simulink model "GNC_integrated_with_guidance"  (R2023a)
settings: Solver=VariableStepAuto  StartTime=0.0  StopTime=200  RelTol=1e-3
undefined symbols (not defined in the file or in its folder): param
libraries: eeGeneralControl x12, simulink_extras x6, SignalEditorBlockLib x1, sharedTrackingLibrary x1
settings Model: Creator=timme  LastModifiedBy=jipva

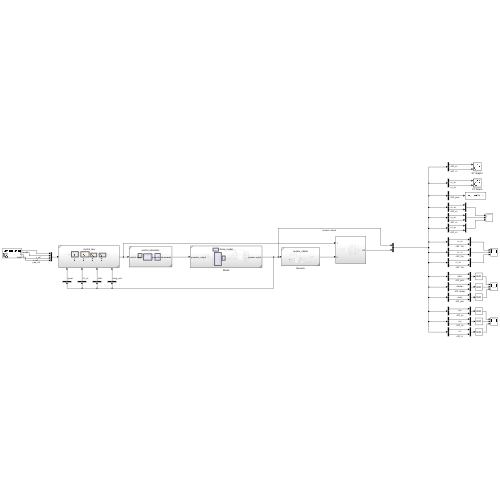
[thumbnail: Simulink's stored preview of the top-level diagram]
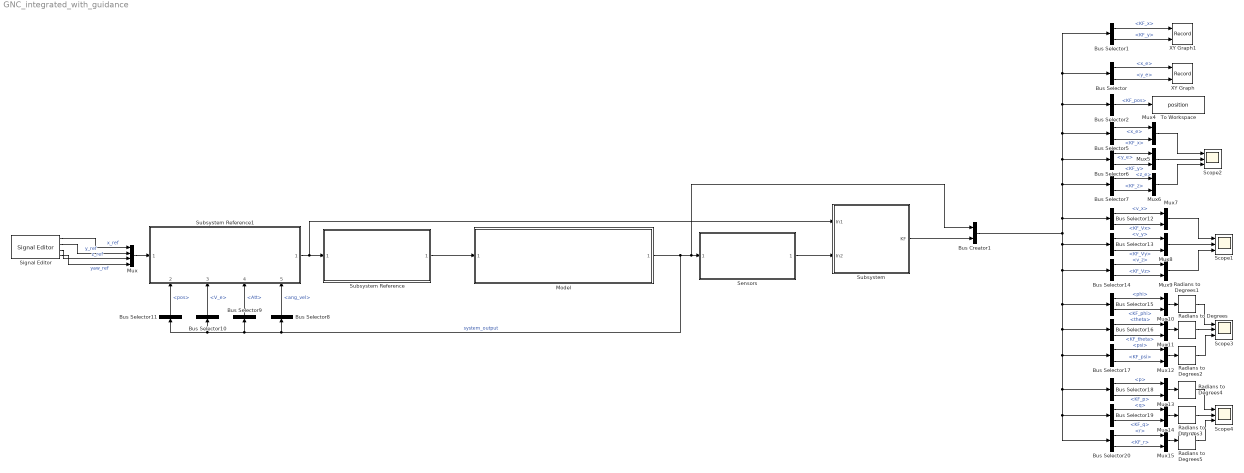
== system GNC_integrated_with_guidance ==
  Bus Creator1 : BusCreator  Inputs=2
  Bus Selector : BusSelector  OutputSignals=system_output.pos.x_e,system_output.pos.y_e
  Bus Selector1 : BusSelector  OutputSignals=KF.KF_pos.KF_x,KF.KF_pos.KF_y
  Bus Selector10 : BusSelector  OutputSignals=V_e
  Bus Selector11 : BusSelector  OutputSignals=pos
  Bus Selector12 : BusSelector  OutputSignals=system_output.V_e.v_x,KF.KF_vel.KF_Vx
  Bus Selector13 : BusSelector  OutputSignals=system_output.V_e.v_y,KF.KF_vel.KF_Vy
  Bus Selector14 : BusSelector  OutputSignals=system_output.V_e.v_z,KF.KF_vel.KF_Vz
  Bus Selector15 : BusSelector  OutputSignals=system_output.Att.phi,KF.KF_att.KF_phi
  Bus Selector16 : BusSelector  OutputSignals=system_output.Att.theta,KF.KF_att.KF_theta
  Bus Selector17 : BusSelector  OutputSignals=system_output.Att.psi,KF.KF_att.KF_psi
  Bus Selector18 : BusSelector  OutputSignals=system_output.ang_vel.p,KF.KF_omega.KF_p
  Bus Selector19 : BusSelector  OutputSignals=system_output.ang_vel.q,KF.KF_omega.KF_q
  Bus Selector2 : BusSelector  OutputSignals=KF.KF_pos
  Bus Selector20 : BusSelector  OutputSignals=system_output.ang_vel.r,KF.KF_omega.KF_r
  Bus Selector5 : BusSelector  OutputSignals=system_output.pos.x_e,KF.KF_pos.KF_x
  Bus Selector6 : BusSelector  OutputSignals=system_output.pos.y_e,KF.KF_pos.KF_y
  Bus Selector7 : BusSelector  OutputSignals=system_output.pos.z_e,KF.KF_pos.KF_z
  Bus Selector8 : BusSelector  OutputSignals=ang_vel
  Bus Selector9 : BusSelector  OutputSignals=Att
  Model : Subsystem  ReferencedSubsystem=drone_model
  Mux : Mux
  Mux{4..15} (12 alike) : Mux  Inputs=2
  Radians to Degrees{,1..5} (6 alike) : simulink_extras/Transformations/Radians to Degrees
  Scope{1..4} (4 alike) : Scope  NumInputPorts=3
  Sensors : Subsystem  ReferencedSubsystem=sensor_model
  Signal Editor : SignalEditorBlockLib/Signal Editor  FileName=C:\Users\jipva\MATLAB\Projects\drone\Detailed design phase\guidance\full_system_reference.mat  ActiveScenario=StandardScenario  ActiveSignal=yaw  IsBus=off  OutputBusObjectStr=Bus: BusObject  SampleTime=param.dt  ZeroCross=off  OutputAfterFinalValue=Setting to zero  Unit=inherit  PreserveSignalName=on  ApplySigPropsToAllScenarios=on
  Subsystem : Subsystem
  Subsystem Reference : Subsystem  ReferencedSubsystem=control_allocation
  Subsystem Reference1 : Subsystem  ReferencedSubsystem=control_law
      settings: PortSchema="{\"entries\":[{\"content\":{\"sides\":[{\"content\":{\"connectorIds\":[\"In1\"]},\"type\":\"ConnectorPlacement.EquallySpacedRectSide\",\"uuid\":\"cbb659e7-d19a-4e68-9ae7-e5e39426296b\"},{\"content\":{\"connectorIds\":[\"Out1\"],\"side\":\"RIGHT\"},\"type\":\"ConnectorPlacement.EquallySpacedRectSide\",\"uuid\":\"c9f08a4e-80d9-41bf-93e6-4cfd11b32426\"},{\"content\":{\"side\":\"TOP\"},\"type\":\"ConnectorPlacement.EquallySpacedRectSide\",\"uuid\":\"8eafc22d-128e-4ca7-9eba-2c3fd299252c\"},{\"content\":{\"connectorIds\":[\"In2\",\"In3\",\"In4\",\"In5\"],\"side\":\"BOTTOM\"},\"type\":\"ConnectorPlacement.EquallySpacedRectSide\",\"uuid\":\"abe1dc09-e6b8-433e-beaf-ba54ebcb4b47\"}]},\"type\":\"ConnectorPlacement.EquallySpacedConnector\",\"uuid\":\"085ffc95-65e8-4235-be8d-72c324b16b8b\"}],\"packageUris\":[\"http://schema.mathworks.com/mf0/Connector/R2020b\"],\"version\":\"1.0\"}"
  To Workspace : ToWorkspace  VariableName=position  SaveFormat=Timeseries  SampleTime=param.dt
  XY Graph : Record  FileSettingsInternal="{\"entries\":[{\"content\":{\"excelSettings\":{\"content\":{},\"type\":\"Streamout.ExcelSettings\"}},\"type\":\"Streamout.FileSettingStorage\",\"uuid\":\"\"}],\"packageUris\":[\"http:\\/\\/schema.mathworks.com\\/mf0\\/streamout_blocks\\/R2020a\"],\"version\":\"1.0\"}"  Layout=[1 1]  SignalsInternal="{\"entries\":[{\"content\":{\"signals\":[{\"content\":{\"blockPath\":[],\"dimensions\":[1],\"domain\":\"\",\"lineColor\":\"#a2142f\",\"plots\":[1],\"port\":1,\"signalID\":16,\"signalName\":\"<x_e>\"},\"type\":\"RecordBlkView.Signal\",\"uuid\":\"\"},{\"content\":{\"blockPath\":[],\"dimensions\":[1],\"domain\":\"\",\"lineColor\":\"#139fff\",\"plots\":[1],\"port\":2,\"signalID\":19,\"signalName\":\"<y_e>\"},\"type\":\"RecordBlkView.Signal\",\"uuid\":\"\"}]},\"type\":\"RecordBlkView.InputSignals\",\"uuid\":\"\"}],\"packageUris\":[\"http:\\/\\/schema.mathworks.com\\/mf0\\/streamout_blocks\\/R2020a\"],\"version\":\"1.0\"}"  VisualizationBindings="{\"xyplotplugin\":{\"info\":[{\"series\":[{\"bindingParametersList\":[{\"parameter\":\"X-Axis\",\"signalID\":16,\"signalName\":\"<x_e>\"},{\"parameter\":\"Y-Axis\",\"signalID\":19,\"signalName\":\"<y_e>\"}],\"seriesID\":34649}],\"subplotID\":1}]}}"  CompatibilityTag=XY
  XY Graph1 : Record  FileSettingsInternal="{\"entries\":[{\"content\":{\"excelSettings\":{\"content\":{},\"type\":\"Streamout.ExcelSettings\"}},\"type\":\"Streamout.FileSettingStorage\",\"uuid\":\"\"}],\"packageUris\":[\"http:\\/\\/schema.mathworks.com\\/mf0\\/streamout_blocks\\/R2020a\"],\"version\":\"1.0\"}"  Layout=[1 1]  SignalsInternal="{\"entries\":[{\"content\":{\"signals\":[{\"content\":{\"blockPath\":[],\"dimensions\":[1],\"domain\":\"\",\"lineColor\":\"#a2142f\",\"plots\":[1],\"port\":1,\"signalID\":8,\"signalName\":\"Second-Order Filter3\"},\"type\":\"RecordBlkView.Signal\",\"uuid\":\"\"},{\"content\":{\"blockPath\":[],\"dimensions\":[1],\"domain\":\"\",\"lineColor\":\"#139fff\",\"plots\":[1],\"port\":2,\"signalID\":11,\"signalName\":\"Second-Order Filter4\"},\"type\":\"RecordBlkView.Signal\",\"uuid\":\"\"}]},\"type\":\"RecordBlkView.InputSignals\",\"uuid\":\"\"}],\"packageUris\":[\"http:\\/\\/schema.mathworks.com\\/mf0\\/streamout_blocks\\/R2020a\"],\"version\":\"1.0\"}"  VisualizationBindings="{\"xyplotplugin\":{\"info\":[{\"series\":[{\"bindingParametersList\":[{\"parameter\":\"X-Axis\",\"signalID\":8,\"signalName\":\"Second-Order Filter3\"},{\"parameter\":\"Y-Axis\",\"signalID\":11,\"signalName\":\"Second-Order Filter4\"}],\"seriesID\":35005}],\"subplotID\":1}]}}"  CompatibilityTag=XY
  wires:
  Model/1 -> Bus Creator1/1, Sensors/1, Bus Selector11/1, Bus Selector10/1, Bus Selector9/1, Bus Selector8/1  "system_output"
  Subsystem Reference1/1 -> Subsystem/1(In1), Subsystem Reference/1
  Bus Selector5/1 -> Mux4/1  "<x_e>"
  Bus Selector5/2 -> Mux4/2  "<KF_x>"
  Bus Selector6/1 -> Mux5/1  "<y_e>"
  Bus Selector6/2 -> Mux5/2  "<KF_y>"
  Bus Selector7/2 -> Mux6/2  "<KF_z>"
  Bus Selector7/1 -> Mux6/1  "<z_e>"
  Bus Selector8/1 -> Subsystem Reference1/5  "<ang_vel>"
  Bus Selector9/1 -> Subsystem Reference1/4  "<Att>"
  Bus Selector10/1 -> Subsystem Reference1/3  "<V_e>"
  Bus Selector11/1 -> Subsystem Reference1/2  "<pos>"
  Bus Selector12/2 -> Mux7/2  "<KF_Vx>"
  Bus Selector12/1 -> Mux7/1  "<v_x>"
  Bus Selector13/1 -> Mux8/1  "<v_y>"
  Bus Selector14/2 -> Mux9/2  "<KF_Vz>"
  Bus Selector14/1 -> Mux9/1  "<v_z>"
  Bus Selector13/2 -> Mux8/2  "<KF_Vy>"
  Bus Selector16/2 -> Mux11/2  "<KF_theta>"
  Mux12/1 -> Radians to Degrees2/1
  Mux11/1 -> Radians to Degrees/1
  Bus Selector17/2 -> Mux12/2  "<KF_psi>"
  Bus Selector17/1 -> Mux12/1  "<psi>"
  Bus Selector15/2 -> Mux10/2  "<KF_phi>"
  Mux10/1 -> Radians to Degrees1/1
  Bus Selector15/1 -> Mux10/1  "<phi>"
  Bus Selector16/1 -> Mux11/1  "<theta>"
  Bus Selector19/2 -> Mux14/2  "<KF_q>"
  Bus Selector18/2 -> Mux13/2  "<KF_p>"
  Mux13/1 -> Radians to Degrees4/1
  Bus Selector20/1 -> Mux15/1  "<r>"
  Bus Selector18/1 -> Mux13/1  "<p>"
  Mux15/1 -> Radians to Degrees5/1
  Bus Selector20/2 -> Mux15/2  "<KF_r>"
  Mux14/1 -> Radians to Degrees3/1
  Bus Selector19/1 -> Mux14/1  "<q>"
  Signal Editor/2 -> Mux/2  "y_ref"
  Signal Editor/1 -> Mux/1  "x_ref"
  Signal Editor/3 -> Mux/3  "z_ref"
  Signal Editor/4 -> Mux/4  "yaw_ref"
  Mux/1 -> Subsystem Reference1/1
  Subsystem Reference/1 -> Model/1
  Bus Selector/1 -> XY Graph/1  "<x_e>"
  Bus Selector/2 -> XY Graph/2  "<y_e>"
  Bus Creator1/1 -> Bus Selector13/1, Bus Selector14/1, Bus Selector20/1, Bus Selector19/1, Bus Selector18/1, Bus Selector17/1, Bus Selector16/1, Bus Selector15/1, Bus Selector12/1, Bus Selector7/1, Bus Selector6/1, Bus Selector2/1, Bus Selector1/1, Bus Selector/1, Bus Selector5/1
  Mux5/1 -> Scope2/2
  Mux4/1 -> Scope2/1
  Mux6/1 -> Scope2/3
  Mux8/1 -> Scope1/2
  Mux9/1 -> Scope1/3
  Mux7/1 -> Scope1/1
  Radians to Degrees2/1 -> Scope3/3
  Radians to Degrees1/1 -> Scope3/1
  Radians to Degrees/1 -> Scope3/2
  Radians to Degrees5/1 -> Scope4/3
  Radians to Degrees4/1 -> Scope4/1
  Radians to Degrees3/1 -> Scope4/2
  Bus Selector1/1 -> XY Graph1/1  "<KF_x>"
  Bus Selector1/2 -> XY Graph1/2  "<KF_y>"
  Sensors/1 -> Subsystem/2(In2)
  Subsystem/1(KF) -> Bus Creator1/2
  Bus Selector2/1 -> To Workspace/1  "<KF_pos>"

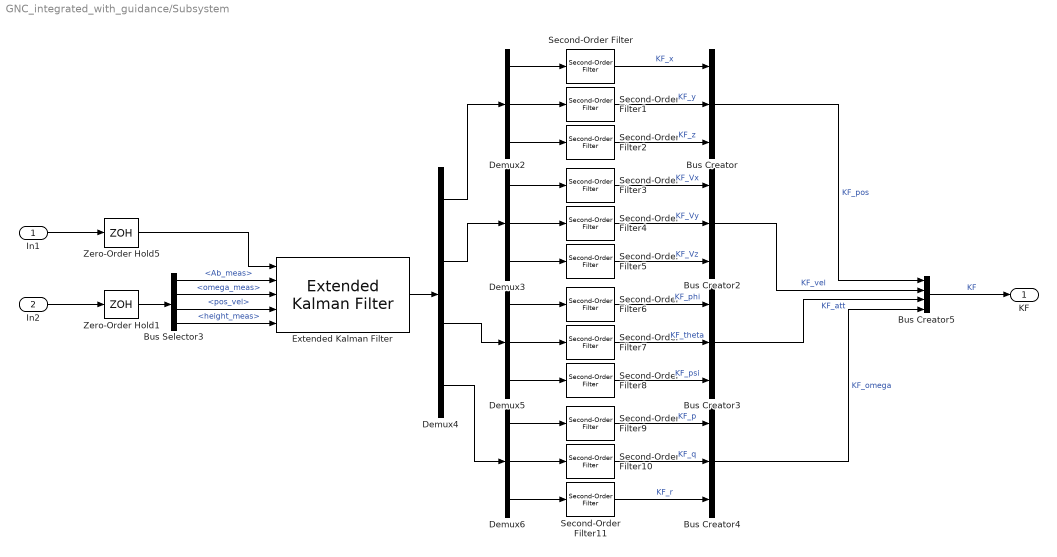
== system GNC_integrated_with_guidance/Subsystem ==
  In1 : Inport
  In2 : Inport  Port=2
  Bus Creator{,2..4} (4 alike) : BusCreator  Inputs=3
  Bus Creator5 : BusCreator  Inputs=4
  Bus Selector3 : BusSelector  OutputSignals=Ab_meas,omega_meas,pos_vel,height_meas
  Demux{2..3,5..6} (4 alike) : Demux  Outputs=3
  Demux4 : Demux
  Extended Kalman Filter : sharedTrackingLibrary/Extended Kalman Filter  StateTransitionFcn=stateTransition  HasStateTransitionJacobianFcn=off  HasAdditiveProcessNoise=Additive  ProcessNoise=10  HasTimeVaryingProcessNoise=off  HasStateTransitionFcnExtraArgument=1  InitialState=zeros(12,1)  InitialStateCovariance=zeros(12)  MeasurementFcn1=accelerometer_model  HasMeasurementJacobianFcn1=off  HasMeasurementEnablePort1=off  HasAdditiveMeasurementNoise1=Additive  MeasurementNoise1=diag([100 100 100])  HasTimeVaryingMeasurementNoise1=off  HasMeasurementFcnExtraArgument1=0  HasMeasurementWrapping1=off  MeasurementFcn2=gyrometer_model  HasMeasurementJacobianFcn2=off  HasMeasurementEnablePort2=off  HasAdditiveMeasurementNoise2=Additive  MeasurementNoise2=eye(3)  HasTimeVaryingMeasurementNoise2=off  HasMeasurementFcnExtraArgument2=0  HasMeasurementWrapping2=off  MeasurementFcn3=GPS_model  HasMeasurementJacobianFcn3=off  HasMeasurementEnablePort3=off  HasAdditiveMeasurementNoise3=Additive  MeasurementNoise3=diag([10 10 100 0.1 0.1 0.1])  HasTimeVaryingMeasurementNoise3=off  HasMeasurementFcnExtraArgument3=0  HasMeasurementWrapping3=off  MeasurementFcn4=Barometer_model  HasMeasurementJacobianFcn4=off  HasMeasurementEnablePort4=off  HasAdditiveMeasurementNoise4=Additive  MeasurementNoise4=0.01  HasTimeVaryingMeasurementNoise4=off  HasMeasurementFcnExtraArgument4=0  HasMeasurementWrapping4=off  MeasurementFcn5=myMeasurementFcn  HasMeasurementJacobianFcn5=off  HasMeasurementEnablePort5=off  HasAdditiveMeasurementNoise5=Additive  MeasurementNoise5=1  HasTimeVaryingMeasurementNoise5=off  HasMeasurementFcnExtraArgument5=0  HasMeasurementWrapping5=off  EnableMultirate=off  StateTransitionFcnSampleTime=1  MeasurementFcn1SampleTime=1  MeasurementFcn2SampleTime=1  MeasurementFcn3SampleTime=1  MeasurementFcn4SampleTime=1  MeasurementFcn5SampleTime=1  UseCurrentEstimator=on  OutputStateCovariance=off  DataType=double  SampleTime=0.01  NumberOfMeasurements=4
  Second-Order Filter{,1..11} (12 alike) : eeGeneralControl/Second-Order Filter  FilterType=Low-pass  fn=10  Zeta=0.707  Ts=param.dt  A0=0  Ph0=0  f0=0  b0=0
      settings: LibrarySourceBlock=ee_sl_lib/General Control/Second-Order Filter
  Zero-Order Hold1 : ZeroOrderHold  SampleTime=param.dt
  Zero-Order Hold5 : ZeroOrderHold  SampleTime=param.dt
  KF : Outport
  wires:
  Demux5/2 -> Second-Order Filter7/1
  Bus Selector3/2 -> Extended Kalman Filter/3  "<omega_meas>"
  Demux6/1 -> Second-Order Filter9/1
  Bus Selector3/3 -> Extended Kalman Filter/4  "<pos_vel>"
  Demux2/3 -> Second-Order Filter2/1
  Zero-Order Hold5/1 -> Extended Kalman Filter/1
  Demux3/1 -> Second-Order Filter3/1
  Zero-Order Hold1/1 -> Bus Selector3/1
  Demux6/2 -> Second-Order Filter10/1
  Demux6/3 -> Second-Order Filter11/1
  Demux5/3 -> Second-Order Filter8/1
  Bus Creator2/1 -> Bus Creator5/2  "KF_vel"
  Bus Creator/1 -> Bus Creator5/1  "KF_pos"
  Demux4/2 -> Demux3/1
  Demux3/3 -> Second-Order Filter5/1
  Demux2/1 -> Second-Order Filter/1
  Bus Creator4/1 -> Bus Creator5/4  "KF_omega"
  Demux4/1 -> Demux2/1
  Demux5/1 -> Second-Order Filter6/1
  Bus Selector3/1 -> Extended Kalman Filter/2  "<Ab_meas>"
  Demux3/2 -> Second-Order Filter4/1
  Bus Selector3/4 -> Extended Kalman Filter/5  "<height_meas>"
  Bus Creator3/1 -> Bus Creator5/3  "KF_att"
  Demux4/4 -> Demux6/1
  In2/1 -> Zero-Order Hold1/1
  Second-Order Filter1/1 -> Bus Creator/2  "KF_y"
  Extended Kalman Filter/1 -> Demux4/1
  Demux4/3 -> Demux5/1
  Bus Creator5/1 -> KF/1  "KF"
  In1/1 -> Zero-Order Hold5/1
  Second-Order Filter/1 -> Bus Creator/1  "KF_x"
  Demux2/2 -> Second-Order Filter1/1
  Second-Order Filter2/1 -> Bus Creator/3  "KF_z"
  Second-Order Filter3/1 -> Bus Creator2/1  "KF_Vx"
  Second-Order Filter4/1 -> Bus Creator2/2  "KF_Vy"
  Second-Order Filter5/1 -> Bus Creator2/3  "KF_Vz"
  Second-Order Filter6/1 -> Bus Creator3/1  "KF_phi"
  Second-Order Filter7/1 -> Bus Creator3/2  "KF_theta"
  Second-Order Filter8/1 -> Bus Creator3/3  "KF_psi"
  Second-Order Filter9/1 -> Bus Creator4/1  "KF_p"
  Second-Order Filter10/1 -> Bus Creator4/2  "KF_q"
  Second-Order Filter11/1 -> Bus Creator4/3  "KF_r"
